simulink model "tvc_lqr_gain_scheduled"  (R2025b)
settings: Solver=VariableStepAuto  StartTime=0.0  StopTime=20  RelTol=1e-3
values from neighbouring files (symbols this model uses):
  A_sys = [ 0, 1, 0, 0, 0, 0 ... (first row only)    [starship_tvc_extended_states.m]
  B_sys = [0, 0, 0, 0; K_phi, -K_phi, 0, 0; 0, 0, 0, 0; 0, 0, Ctp_max, 0; 0, 0, 0, 0; 0, 0, 0, Cty_max]    [starship_tvc_extended_states.m]
  C_sys = eye(6)    [starship_tvc_extended_states.m]
  D_sys = zeros(6, 4)    [starship_tvc_extended_states.m]
  Gain_Index = 1:24    [starship_tvc_extended_states.m]
  K_curr = lqr(A_sys, B_curr, Q, R)    [starship_tvc_extended_states.m]
  K_schedule_data = zeros(length(T_schedule), 24)    [starship_tvc_extended_states.m]
  T_schedule = g * [0.11, 0.43, 0.95, 1.5, 1.91, 2.45, 3.1, 3.5, 3.9, 4.23]    [starship_tvc_extended_states.m]
settings Model: Creator=freak  LastModifiedBy=freak

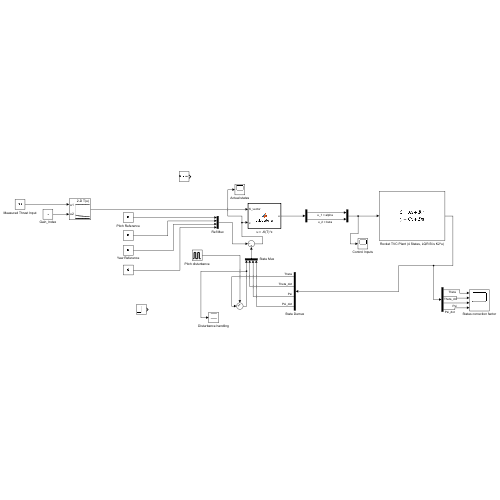
[thumbnail: Simulink's stored preview of the top-level diagram]
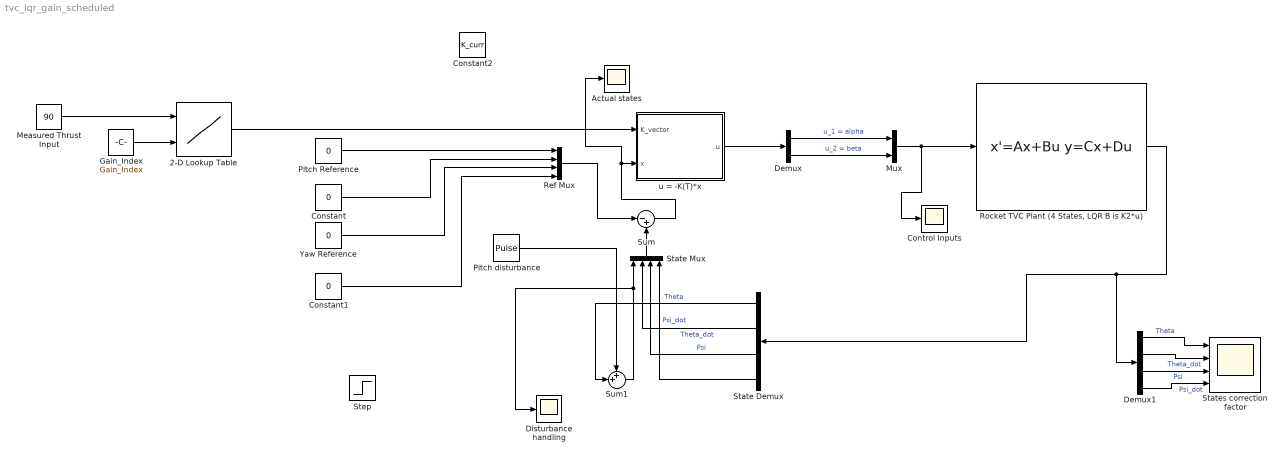
== system tvc_lqr_gain_scheduled ==
  2-D Lookup Table : Lookup_n-D  BreakpointsForDimension1=T_schedule  BreakpointsForDimension2=Gain_Index  IndexSearchMethod=Evenly spaced points  Table=K_schedule_data  InternalRulePriority=Speed  RndMeth=Simplest
      settings: InputPortMap=u0,u1
  Actual states : Scope
      settings: ActiveDisplayYMinimum=-0.46880516298147618  ActiveDisplayYMaximum=0.45896834599975539
  Constant : Constant  Value=0
  Constant1 : Constant  Value=0
  Constant2 : Constant  Value=K_curr
  Control Inputs : Scope
      settings: ActiveDisplayYMinimum=-2.9579809113570303  ActiveDisplayYMaximum=2.9231355464726687
  Demux : Demux  Outputs=2
  Demux1 : Demux
  Disturbance handling : Scope
      settings: ActiveDisplayYMinimum=-0.11123898226754711  ActiveDisplayYMaximum=0.11235988691861634  DataLoggingVariableName=ScopeData3
  Gain_Index : Constant  Value=Gain_Index
  Measured Thrust Input : Constant  Value=90
  Mux : Mux  Inputs=2
  Pitch Reference : Constant  Value=0
  Pitch disturbance : DiscretePulseGenerator  PulseType=Time based  Amplitude=0.09  Period=20  PulseWidth=30  PhaseDelay=2
  Ref Mux : Mux
  "Rocket TVC Plant (4 States, LQR B is K2*u)" : StateSpace  A=A_sys  B=B_sys  C=C_sys  D=D_sys  InitialCondition=0  ContinuousStateAttributes={'theta','theta_dot','psi','psi_dot'}
  State Demux : Demux
  State Mux : Mux
  States correction factor : Scope  NumInputPorts=4
      settings: ActiveDisplayYMinimum=-15.985055648407965  ActiveDisplayYMaximum=13.775552616374139  DataLoggingVariableName=ScopeData2
  Step : Step  Time=3  After=0.09  SampleTime=0
  Sum : Sum  Inputs=|-+
  Sum1 : Sum  Inputs=++|
  Yaw Reference : Constant  Value=0
  u = -K(T)*x : MATLAB Function  TreatAsAtomicUnit=on
  wires:
  "Rocket TVC Plant (4 States, LQR B is K2*u)"/1 -> Demux1/1, State Demux/1
  State Demux/4 -> State Mux/4  "Psi_dot"
  Measured Thrust Input/1 -> 2-D Lookup Table/1
  Gain_Index/1 -> 2-D Lookup Table/2
  u = -K(T)*x/1(u) -> Demux/1
  Constant/1 -> Ref Mux/2
  Yaw Reference/1 -> Ref Mux/3
  Constant1/1 -> Ref Mux/4
  State Mux/1 -> Sum/2
  Sum/1 -> Actual states/1, u = -K(T)*x/2(x)
  State Demux/2 -> State Mux/2  "Theta_dot"
  State Demux/3 -> State Mux/3  "Psi"
  Ref Mux/1 -> Sum/1
  Pitch Reference/1 -> Ref Mux/1
  Mux/1 -> Control Inputs/1, "Rocket TVC Plant (4 States, LQR B is K2*u)"/1
  Demux/2 -> Mux/2  "u_2 = beta"
  Demux/1 -> Mux/1  "u_1 = alpha"
  Sum1/1 -> State Mux/1, Disturbance handling/1
  Demux1/1 -> States correction factor/1  "Theta"
  Demux1/2 -> States correction factor/2  "Theta_dot"
  Demux1/3 -> States correction factor/3  "Psi"
  Demux1/4 -> States correction factor/4  "Psi_dot"
  State Demux/1 -> Sum1/2  "Theta"
  Pitch disturbance/1 -> Sum1/1
  2-D Lookup Table/1 -> u = -K(T)*x/1(K_vector)

== matlab function tvc_lqr_gain_scheduled/u = -K(T)*x ==
  data: K_vector input; u output; x input
function u = calculate_u(K_vector, x)
% u = -K * x; 
% Inputs:
%   K_vector: 8x1 or 1x8 vector of gains from Lookup Table
%   x: 4x1 State vector [theta; theta_dot; psi; psi_dot]

% Reshape vector back into 2x4 Gain Matrix that is equal to K_curr
K = reshape(K_vector, 2, 4)
% K = K_vector;

% Calculate Control Law
u = -K * x;
